simulink model "P_k"  (R2024b)
settings: Solver=FixedStepAuto  StartTime=0.0  StopTime=10  FixedStep=1  RelTol=1e-3
undefined symbols (not defined in the file): I_a
settings Model: Creator=54238  LastModifiedBy=54238

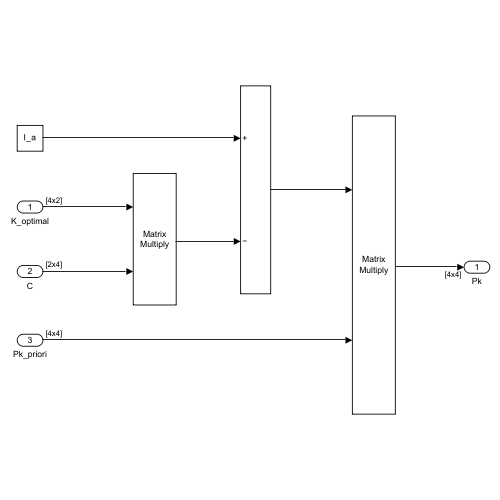
[thumbnail: Simulink's stored preview of the top-level diagram]
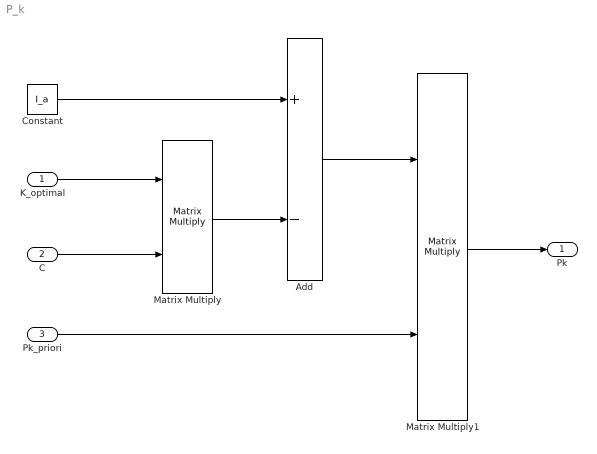
== system P_k ==
  K_optimal : Inport  PortDimensions=[4,2]
  C : Inport  Port=2  PortDimensions=[2,4]
  Pk_priori : Inport  Port=3  PortDimensions=[4,4]
  Add : Sum  Inputs=+-
  Constant : Constant  Value=I_a
  Matrix Multiply : Product  Multiplication=Matrix(*)
  Matrix Multiply1 : Product  Multiplication=Matrix(*)
  Pk : Outport  PortDimensions=[4,4]
  wires:
  K_optimal/1 -> Matrix Multiply/1
  C/1 -> Matrix Multiply/2
  Constant/1 -> Add/1
  Matrix Multiply/1 -> Add/2
  Add/1 -> Matrix Multiply1/1
  Pk_priori/1 -> Matrix Multiply1/2
  Matrix Multiply1/1 -> Pk/1
